simulink model "MAS_FOC"  (R2024b)
settings: Solver=VariableStepAuto  StartTime=0.0  StopTime=3  RelTol=1e-3
InitFcn:
  | init_mas
values from neighbouring files (symbols this model uses):
  Kphi = 15.21    [init_mas.m]
  Kq = 1.65    [init_mas.m]
  Tq = 0.0165    [init_mas.m]
libraries: slpidlib x2
settings Model: Creator=firas  LastModifiedBy=firas

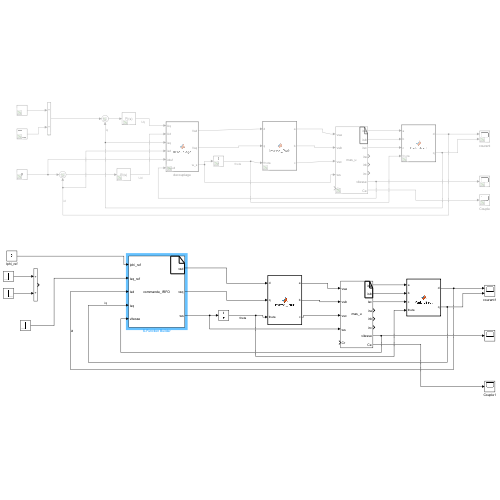
[thumbnail: Simulink's stored preview of the top-level diagram]
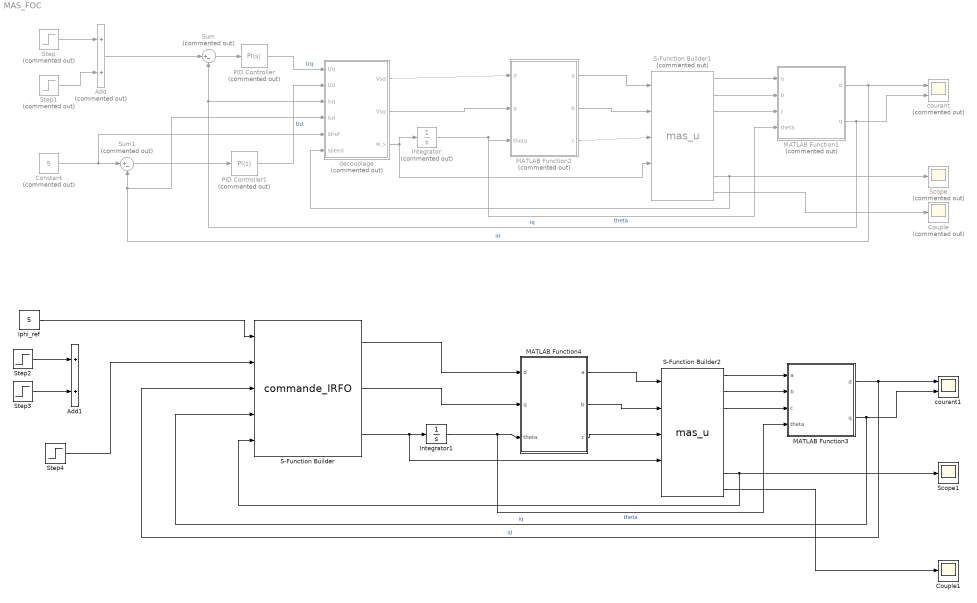
== system MAS_FOC ==
  Add : Sum  Commented=on
  Add1 : Sum
  Constant : Constant  Commented=on  Value=5
  Couple : Scope  Commented=on
  Couple1 : Scope
  Integrator : Integrator  Commented=on
  Integrator1 : Integrator
  Iphi_ref : Constant  Value=5
  MATLAB Function1 : MATLAB Function  Commented=on  TreatAsAtomicUnit=on
  MATLAB Function2 : MATLAB Function  Commented=on  TreatAsAtomicUnit=on
  MATLAB Function3 : MATLAB Function  TreatAsAtomicUnit=on
  MATLAB Function4 : MATLAB Function  TreatAsAtomicUnit=on
  PID Controller : slpidlib/PID Controller  Commented=on  Controller=PI  Form=Parallel  TimeDomain=Continuous-time  UseExternalTs=off  SampleTime=-1  IntegratorMethod=Forward Euler  FilterMethod=Forward Euler  ControllerParametersSource=internal  P=Kq  I=Kq/Tq  UseKiTs=off  D=0  UseExternalDerivativeSource=off  N=100  UseFilter=on  TunerSelectOption=Transfer Function Based (PID Tuner App)  InitialConditionSource=internal  InitialConditionForIntegrator=0  InitialConditionForFilter=0  DifferentiatorICPrevScaledInput=0  ExternalReset=none  TrackingMode=off  Kt=1  LimitOutput=off  SatLimitsSource=internal  UpperSaturationLimit=inf  LowerSaturationLimit=-inf  LinearizeAsGain=on  AntiWindupMode=none  Kb=1  LimitIntegrator=off  UpperIntegratorSaturationLimit=inf  LowerIntegratorSaturationLimit=-inf  POutMin=[]  POutMax=[]  IOutMin=[]  IOutMax=[]  DOutMin=[]  DOutMax=[]  NOutMin=[]  NOutMax=[]  SumOutMin=[]  SumOutMax=[]  SaturationOutMin=[]  SaturationOutMax=[]  PParamMin=[]  PParamMax=[]  IParamMin=[]  IParamMax=[]  DParamMin=[]  DParamMax=[]  NParamMin=[]  NParamMax=[]  KbParamMin=[]  KbParamMax=[]  KtParamMin=[]  KtParamMax=[]  KbOutMin=[]  KbOutMax=[]  KtOutMin=[]  KtOutMax=[]  IntegratorOutMin=[]  IntegratorOutMax=[]  FilterOutMin=[]  FilterOutMax=[]  SumI1OutMin=[]  SumI1OutMax=[]  SumI2OutMin=[]  SumI2OutMax=[]  SumI3OutMin=[]  SumI3OutMax=[]  SumI4OutMin=[]  SumI4OutMax=[]  SumDOutMin=[]  SumDOutMax=[]  DifferentiatorOutMin=[]  DifferentiatorOutMax=[]  FilterDiffOutCoefMin=[]  FilterDiffOutCoefMax=[]  ReciprocalOutMin=[]  ReciprocalOutMax=[]  SumDenOutMin=[]  SumDenOutMax=[]  SumNumOutMin=[]  SumNumOutMax=[]  DivideOutMin=[]  DivideOutMax=[]  UdiffTsProdOutMin=[]  UdiffTsProdOutMax=[]  NTsProdOutMin=[]  NTsProdOutMax=[]  UintegralTsProdOutMin=[]  UintegralTsProdOutMax=[]  UngainTsProdOutMin=[]  UngainTsProdOutMax=[]  ClampingZeroOutDataTypeStr=Inherit: Inherit via back propagation  ClampingZeroOutMin=[]  ClampingZeroOutMax=[]  FilterDenConstantOutDataTypeStr=Inherit: Inherit via back propagation  FilterDenConstantOutMin=[]  FilterDenConstantOutMax=[]  PCopyOutDataTypeStr=Inherit: Inherit via back propagation  PCopyOutMin=[]  PCopyOutMax=[]  NCopyOutDataTypeStr=Inherit: Inherit via back propagation  NCopyOutMin=[]  NCopyOutMax=[]  IntegratorContinuousStateAttributes=''  IntegratorStateMustResolveToSignalObject=off  IntegratorRTWStateStorageClass=Auto  FilterContinuousStateAttributes=''  FilterStateMustResolveToSignalObject=off  FilterRTWStateStorageClass=Auto  ParallelPVariant=InternalParameters  IdealPVariant=Disabled  IVariant=InternalParameters  DVariant=Disabled  IntegratorVariant=Continuous  SatVariant=Disabled  AWVariant=Passthrough  PCopyVariant=Disabled  TRVariant=Disabled  FdbkBlocksVariant=Forward  IdealPFdbkVariant=Disabled  SatFdbkVariant=Disabled  DerivativeFilterVariant=Disabled  NVariant=Disabled  NCopyVariant=Disabled_SignalSpec  FilterICVariant=Disabled  IntegratorICVariant=InternalICs  ExternalResetVariant=Disabled  TRSumVariant=Passthrough  SumFdbkVariant=Disabled  SumVariant=Sum_PI  TsampFilterVariant=InternalTs  TsampNgainVariant=Passthrough  TsampIntegralVariant=Disabled_SignalSpec  ExternalSaturationOutDataTypeStr=Inherit: Same as second input  DerivativeSourceVariant=Disabled  PreIntVariant=InternalPreInt
  PID Controller1 : slpidlib/PID Controller  Commented=on  Controller=PI  Form=Parallel  TimeDomain=Continuous-time  UseExternalTs=off  SampleTime=-1  IntegratorMethod=Forward Euler  FilterMethod=Forward Euler  ControllerParametersSource=internal  P=Kphi  I=Kphi/Tq  UseKiTs=off  D=0  UseExternalDerivativeSource=off  N=100  UseFilter=on  TunerSelectOption=Transfer Function Based (PID Tuner App)  InitialConditionSource=internal  InitialConditionForIntegrator=0  InitialConditionForFilter=0  DifferentiatorICPrevScaledInput=0  ExternalReset=none  TrackingMode=off  Kt=1  LimitOutput=off  SatLimitsSource=internal  UpperSaturationLimit=inf  LowerSaturationLimit=-inf  LinearizeAsGain=on  AntiWindupMode=none  Kb=1  LimitIntegrator=off  UpperIntegratorSaturationLimit=inf  LowerIntegratorSaturationLimit=-inf  POutMin=[]  POutMax=[]  IOutMin=[]  IOutMax=[]  DOutMin=[]  DOutMax=[]  NOutMin=[]  NOutMax=[]  SumOutMin=[]  SumOutMax=[]  SaturationOutMin=[]  SaturationOutMax=[]  PParamMin=[]  PParamMax=[]  IParamMin=[]  IParamMax=[]  DParamMin=[]  DParamMax=[]  NParamMin=[]  NParamMax=[]  KbParamMin=[]  KbParamMax=[]  KtParamMin=[]  KtParamMax=[]  KbOutMin=[]  KbOutMax=[]  KtOutMin=[]  KtOutMax=[]  IntegratorOutMin=[]  IntegratorOutMax=[]  FilterOutMin=[]  FilterOutMax=[]  SumI1OutMin=[]  SumI1OutMax=[]  SumI2OutMin=[]  SumI2OutMax=[]  SumI3OutMin=[]  SumI3OutMax=[]  SumI4OutMin=[]  SumI4OutMax=[]  SumDOutMin=[]  SumDOutMax=[]  DifferentiatorOutMin=[]  DifferentiatorOutMax=[]  FilterDiffOutCoefMin=[]  FilterDiffOutCoefMax=[]  ReciprocalOutMin=[]  ReciprocalOutMax=[]  SumDenOutMin=[]  SumDenOutMax=[]  SumNumOutMin=[]  SumNumOutMax=[]  DivideOutMin=[]  DivideOutMax=[]  UdiffTsProdOutMin=[]  UdiffTsProdOutMax=[]  NTsProdOutMin=[]  NTsProdOutMax=[]  UintegralTsProdOutMin=[]  UintegralTsProdOutMax=[]  UngainTsProdOutMin=[]  UngainTsProdOutMax=[]  ClampingZeroOutDataTypeStr=Inherit: Inherit via back propagation  ClampingZeroOutMin=[]  ClampingZeroOutMax=[]  FilterDenConstantOutDataTypeStr=Inherit: Inherit via back propagation  FilterDenConstantOutMin=[]  FilterDenConstantOutMax=[]  PCopyOutDataTypeStr=Inherit: Inherit via back propagation  PCopyOutMin=[]  PCopyOutMax=[]  NCopyOutDataTypeStr=Inherit: Inherit via back propagation  NCopyOutMin=[]  NCopyOutMax=[]  IntegratorContinuousStateAttributes=''  IntegratorStateMustResolveToSignalObject=off  IntegratorRTWStateStorageClass=Auto  FilterContinuousStateAttributes=''  FilterStateMustResolveToSignalObject=off  FilterRTWStateStorageClass=Auto  ParallelPVariant=InternalParameters  IdealPVariant=Disabled  IVariant=InternalParameters  DVariant=Disabled  IntegratorVariant=Continuous  SatVariant=Disabled  AWVariant=Passthrough  PCopyVariant=Disabled  TRVariant=Disabled  FdbkBlocksVariant=Forward  IdealPFdbkVariant=Disabled  SatFdbkVariant=Disabled  DerivativeFilterVariant=Disabled  NVariant=Disabled  NCopyVariant=Disabled_SignalSpec  FilterICVariant=Disabled  IntegratorICVariant=InternalICs  ExternalResetVariant=Disabled  TRSumVariant=Passthrough  SumFdbkVariant=Disabled  SumVariant=Sum_PI  TsampFilterVariant=InternalTs  TsampNgainVariant=Passthrough  TsampIntegralVariant=Disabled_SignalSpec  ExternalSaturationOutDataTypeStr=Inherit: Same as second input  DerivativeSourceVariant=Disabled  PreIntVariant=InternalPreInt
  S-Function Builder : S-Function  FunctionName=commande_IRFO  SFunctionModules=commande_IRFO_wrapper.c  SFunctionDeploymentMode=off  EnableBusSupport=off  mask(S-Function Builder){}
      mask help: Simulink:masks:SFunctionBuilder_MD
      mask init:
      | val = [[.9  0.75 0.75 1 1 .9 .9 1]',[1 1 0.75 0.75 .9 .9 1 .9]'];try , sys = get_param(gcb,'SfunBuilderFcnName');if isempty(sys), sys = get_param(gcb,'FunctionName'); end,catch, sys = get_param(gcb,'FunctionName'); end
      settings: CopyFcn=set_param(gcbh,'LinkStatus','none')  OpenFcn=sfunctionwizard(gcbh)
      mask Display:
      | plot(val(:,1),val(:,2))
      | disp(sys)
      | port_label('input',1,sprintf('%s', 'iphi\_ref'),'interpreter','tex')
      | port_label('input',2,sprintf('%s', 'isq\_ref'),'interpreter','tex')
      | port_label('input',3,sprintf('%s', 'isd'),'interpreter','tex')
      | port_label('input',4,sprintf('%s', 'isq'),'interpreter','tex')
      | port_label('input',5,sprintf('%s', 'vitesse'),'interpreter','tex')
      | port_label('output',1,sprintf('%s', 'vsd'),'interpreter','tex')
      | port_label('output',2,sprintf('%s', 'vsq'),'interpreter','tex')
      | port_label('output',3,sprintf('%s', 'ws'),'interpreter','tex')
  S-Function Builder1 : S-Function  Commented=on  FunctionName=mas_u  SFunctionModules=mas_u_wrapper.c  SFunctionDeploymentMode=off  EnableBusSupport=off  mask(S-Function Builder){}
      mask help: Simulink:masks:SFunctionBuilder_MD
      mask init: same as MAS_FOC/S-Function Builder
      settings: CopyFcn=set_param(gcbh,'LinkStatus','none')  OpenFcn=sfunctionwizard(gcbh)
      mask Display:
      | plot(val(:,1),val(:,2))
      | disp(sys)
      | port_label('input',1,sprintf('%s', 'vsa'),'interpreter','tex')
      | port_label('input',2,sprintf('%s', 'vsb'),'interpreter','tex')
      | port_label('input',3,sprintf('%s', 'vsc'),'interpreter','tex')
      | port_label('input',4,sprintf('%s', 'ws'),'interpreter','tex')
      | port_label('input',5,sprintf('%s', 'Cr'),'interpreter','tex')
      | port_label('output',1,sprintf('%s', 'isa'),'interpreter','tex')
      | port_label('output',2,sprintf('%s', 'isb'),'interpreter','tex')
      | port_label('output',3,sprintf('%s', 'isc'),'interpreter','tex')
      | port_label('output',4,sprintf('%s', 'ira'),'interpreter','tex')
      | port_label('output',5,sprintf('%s', 'irb'),'interpreter','tex')
      | port_label('output',6,sprintf('%s', 'irc'),'interpreter','tex')
      | port_label('output',7,sprintf('%s', 'vitesse'),'interpreter','tex')
      | port_label('output',8,sprintf('%s', 'Ce'),'interpreter','tex')
  S-Function Builder2 : S-Function  FunctionName=mas_u  SFunctionModules=mas_u_wrapper.c  SFunctionDeploymentMode=off  EnableBusSupport=off  mask(S-Function Builder){}
      mask help: Simulink:masks:SFunctionBuilder_MD
      mask init: same as MAS_FOC/S-Function Builder
      settings: CopyFcn=set_param(gcbh,'LinkStatus','none')  OpenFcn=sfunctionwizard(gcbh)
      mask Display:
      | plot(val(:,1),val(:,2))
      | disp(sys)
      | port_label('input',1,sprintf('%s', 'vsa'),'interpreter','tex')
      | port_label('input',2,sprintf('%s', 'vsb'),'interpreter','tex')
      | port_label('input',3,sprintf('%s', 'vsc'),'interpreter','tex')
      | port_label('input',4,sprintf('%s', 'ws'),'interpreter','tex')
      | port_label('input',5,sprintf('%s', 'Cr'),'interpreter','tex')
      | port_label('output',1,sprintf('%s', 'isa'),'interpreter','tex')
      | port_label('output',2,sprintf('%s', 'isb'),'interpreter','tex')
      | port_label('output',3,sprintf('%s', 'isc'),'interpreter','tex')
      | port_label('output',4,sprintf('%s', 'ira'),'interpreter','tex')
      | port_label('output',5,sprintf('%s', 'irb'),'interpreter','tex')
      | port_label('output',6,sprintf('%s', 'irc'),'interpreter','tex')
      | port_label('output',7,sprintf('%s', 'vitesse'),'interpreter','tex')
      | port_label('output',8,sprintf('%s', 'Ce'),'interpreter','tex')
  Scope : Scope  Commented=on
  Scope1 : Scope
  Step : Step  Commented=on  Time=5  After=8  SampleTime=0
  Step1 : Step  Commented=on  Time=10  After=-4  SampleTime=0
  Step2 : Step  Time=5  After=8  SampleTime=0
  Step3 : Step  Time=10  After=-4  SampleTime=0
  Step4 : Step  Time=2  After=5  SampleTime=0
  Sum : Sum  Commented=on  Inputs=|+-
  Sum1 : Sum  Commented=on  Inputs=|+-
  courant : Scope  Commented=on  NumInputPorts=2
  courant1 : Scope  NumInputPorts=2
  decouplage : MATLAB Function  Commented=on  TreatAsAtomicUnit=on
  wires:
  S-Function Builder1/1 -> MATLAB Function1/1(a)
  S-Function Builder1/2 -> MATLAB Function1/2(b)
  S-Function Builder1/3 -> MATLAB Function1/3(c)
  MATLAB Function1/1(d) -> decouplage/4(isd), Sum1/2, courant/1  "id"
  MATLAB Function1/2(q) -> Sum/2, decouplage/3(isq), courant/2  "iq"
  S-Function Builder1/8 -> Couple/1
  MATLAB Function2/1(a) -> S-Function Builder1/1
  MATLAB Function2/2(b) -> S-Function Builder1/2
  MATLAB Function2/3(c) -> S-Function Builder1/3
  Add/1 -> Sum/1
  Constant/1 -> decouplage/5(idref), Sum1/1
  Sum/1 -> PID Controller/1
  Sum1/1 -> PID Controller1/1
  PID Controller/1 -> decouplage/1(Uq)  "Uq"
  PID Controller1/1 -> decouplage/2(Ud)  "Ud"
  Integrator/1 -> MATLAB Function1/4(theta), MATLAB Function2/3(theta)  "theta"
  decouplage/3(w_s) -> Integrator/1, S-Function Builder1/4
  decouplage/2(Vsq) -> MATLAB Function2/2(q)
  decouplage/1(Vsd) -> MATLAB Function2/1(d)
  S-Function Builder1/7 -> decouplage/6(speed), Scope/1
  Step1/1 -> Add/2
  Step/1 -> Add/1
  S-Function Builder2/7 -> S-Function Builder/5, Scope1/1
  S-Function Builder/1 -> MATLAB Function4/1(d)
  S-Function Builder/2 -> MATLAB Function4/2(q)
  S-Function Builder/3 -> S-Function Builder2/4, Integrator1/1
  Integrator1/1 -> MATLAB Function4/3(theta), MATLAB Function3/4(theta)  "theta"
  MATLAB Function4/3(c) -> S-Function Builder2/3
  MATLAB Function4/2(b) -> S-Function Builder2/2
  MATLAB Function4/1(a) -> S-Function Builder2/1
  S-Function Builder2/8 -> Couple1/1
  MATLAB Function3/2(q) -> courant1/2, S-Function Builder/4  "iq"
  MATLAB Function3/1(d) -> courant1/1, S-Function Builder/3  "id"
  S-Function Builder2/3 -> MATLAB Function3/3(c)
  S-Function Builder2/2 -> MATLAB Function3/2(b)
  S-Function Builder2/1 -> MATLAB Function3/1(a)
  Step2/1 -> Add1/1
  Step3/1 -> Add1/2
  Iphi_ref/1 -> S-Function Builder/1
  Step4/1 -> S-Function Builder/2

== matlab function MAS_FOC/MATLAB Function1 ==
  data: a input; d output; b input; c input; theta input; q output
function [d,q] = Park_direct(a,b,c,theta)
    
     d = sqrt(2/3)*[cos(theta),cos(theta-2*pi/3),cos(theta+2*pi/3)]*[a;b;c];
     q = sqrt(2/3)*[-sin(theta),-sin(theta -2*pi/3),-sin(theta +2*pi/3)]*[a ; b ; c];
    
end

== matlab function MAS_FOC/decouplage ==
  data: Uq input; Vsd output; Ud input; isq input; isd input; idref input; speed input; Vsq output; w_s output
function [Vsd,Vsq,w_s] = decouplage(Uq, Ud , isq,isd,idref,speed)
    Tr =0.153;
    p=2;
    sig = 0.066;
    Ls = 0.25;

    w_s = isq/(Tr*idref) +p*speed;

    ed= -sig*Ls*w_s*isq;
    eq =sig*Ls*w_s*isd+(1-sig)*Ls*w_s*isd;

    Vsd = Ud+ed;
    Vsq = Uq+eq;

end

== matlab function MAS_FOC/MATLAB Function2 ==
  data: d input; a output; q input; theta input; b output; c output
function [a,b,c] = inverse_Park(d,q,theta)
    a = sqrt(2/3)*[cos(theta) -sin(theta)]*[d;q];
    b = sqrt(2/3)*[cos(theta-2*pi/3) -sin(theta-2*pi/3)]*[d;q];
    c = sqrt(2/3)*[cos(theta+2*pi/3) -sin(theta+2*pi/3)]*[d;q];
end

== matlab function MAS_FOC/MATLAB Function3 ==
  data: a input; d output; b input; c input; theta input; q output
function [d,q] = Park_direct(a,b,c,theta)
    
     d = sqrt(2/3)*[cos(theta),cos(theta-2*pi/3),cos(theta+2*pi/3)]*[a;b;c];
     q = sqrt(2/3)*[-sin(theta),-sin(theta -2*pi/3),-sin(theta +2*pi/3)]*[a ; b ; c];
    
end

== matlab function MAS_FOC/MATLAB Function4 ==
  data: d input; a output; q input; theta input; b output; c output
function [a,b,c] = inverse_Park(d,q,theta)
    a = sqrt(2/3)*[cos(theta) -sin(theta)]*[d;q];
    b = sqrt(2/3)*[cos(theta-2*pi/3) -sin(theta-2*pi/3)]*[d;q];
    c = sqrt(2/3)*[cos(theta+2*pi/3) -sin(theta+2*pi/3)]*[d;q];
end
